simulink model "mc_att_control_xyk"  (R2024b)
settings: Solver=FixedStepAuto  StartTime=0.0  StopTime=10.0  RelTol=1e-3
undefined symbols (not defined in the file or in its folder): AIRMODE_ROLL_PITCH_YAW, deg, DiscIntNeverNeededParam, MC_ACRO_EXPO, MC_ACRO_EXPO_Y, MC_ACRO_P_MAX, MC_ACRO_R_MAX, MC_ACRO_SUPEXPO, MC_ACRO_SUPEXPOY, MC_ACRO_Y_MAX, MC_AIRMODE, MC_BAT_SCALE_EN, MC_MAN_TILT_TAU, MC_PITCH_P, MC_PITCHRATE_D, MC_PITCHRATE_FF, MC_PITCHRATE_I, MC_PITCHRATE_K, MC_PITCHRATE_MAX, MC_PITCHRATE_P, MC_PR_INT_LIM, MC_ROLL_P, MC_ROLLRATE_D, MC_ROLLRATE_FF, MC_ROLLRATE_I, MC_ROLLRATE_K, MC_ROLLRATE_MAX, MC_ROLLRATE_P, MC_RR_INT_LIM, MC_YAW_P, MC_YAW_WEIGHT, MC_YAWRATE_D, MC_YAWRATE_FF, MC_YAWRATE_I, MC_YAWRATE_K, MC_YAWRATE_MAX, MC_YAWRATE_P, MC_YR_INT_LIM, MPC_MAN_TILT_MAX, MPC_MAN_Y_MAX, MPC_MANTHR_MIN, MPC_THR_CURVE, MPC_THR_HOVER, MPC_THR_MAX, param_mpc_thr_hover, param_mpc_thr_max, rad, s, VEHICLE_TYPE_ROTARY_WING
libraries: simulink x22, aerolibutil x11, sharedtransform x4, aerolibconvert2 x3, vrlib x2, sharedutil x1
(part 2 of 2)

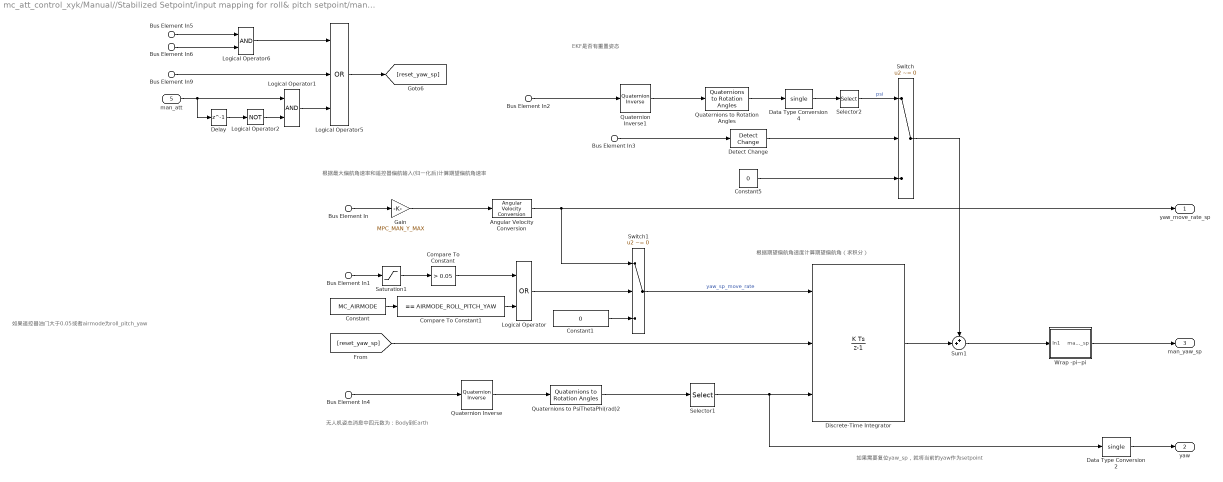
== system mc_att_control_xyk/Manual//Stabilized Setpoint/input mapping for roll& pitch setpoint/man_yaw_sp ==
  note: 无人机姿态消息中四元数为：Body到Earth
  note: 根据期望偏航角速度计算期望偏航角（求积分）
  note: 根据最大偏航角速率和遥控器偏航输入(归一化后)计算期望偏航角速率
  note: 如果遥控器油门大于0.05或者airmode为roll_pitch_yaw
  note: EKF是否有重置姿态
  note: 如果需要复位yaw_sp，就将当前的yaw作为setpoint
  Bus Element In2 : Inport  PortName=att  Element=delta_q_reset
  Bus Element In3 : Inport  PortName=att  Element=quat_reset_counter
  Bus Element In4 : Inport  PortName=att  Element=q
  Bus Element In : Inport  Port=2  PortName=manual_setpoint  Element=r
  Bus Element In1 : Inport  Port=2  PortName=manual_setpoint  Element=z
  Bus Element In5 : Inport  Port=3  PortName=vehicle_status  Element=is_vtol
  Bus Element In6 : Inport  Port=3  PortName=vehicle_status  Element=in_transition_mode
  Bus Element In9 : Inport  Port=4  PortName=vehicle_land_detected  Element=landed
  man_att : Inport  Port=5
  Angular Velocity Conversion : aerolibconvert2/Angular Velocity Conversion  IU=deg/s  OU=rad/s
  Compare To Constant : simulink/Logic and Bit Operations/Compare To Constant  relop=>  const=0.05  OutDataTypeStr=boolean
  Compare To Constant1 : simulink/Logic and Bit Operations/Compare To Constant  relop===  const=AIRMODE_ROLL_PITCH_YAW  OutDataTypeStr=boolean
  Constant : Constant  Value=MC_AIRMODE
  Constant1 : Constant  Value=0  OutDataTypeStr=single
  Constant5 : Constant  Value=0  OutDataTypeStr=single
  Data Type Conversion2 : DataTypeConversion  OutDataTypeStr=single  SaturateOnIntegerOverflow=off  RndMeth=Floor
  Data Type Conversion4 : DataTypeConversion  OutDataTypeStr=single  SaturateOnIntegerOverflow=off  RndMeth=Floor
  Delay : Delay  DelayLength=1  InitialCondition=0
  Detect Change : simulink/Logic and Bit Operations/Detect Change  vinit=0  OutDataTypeStr=boolean
  Discrete-Time Integrator : DiscreteIntegrator  ExternalReset=level  InitialConditionSource=external  SampleTime=-1  LimitOutput=on  UpperSaturationLimit=pi  LowerSaturationLimit=-pi  ICPrevOutput=DiscIntNeverNeededParam  ICPrevScaledInput=DiscIntNeverNeededParam
  Gain : Gain  Gain=MPC_MAN_Y_MAX
      settings: AttributesFormatString=%<Gain>
  Logical Operator : Logic  Operator=OR  AllPortsSameDT=off  OutDataTypeStr=boolean
  Logical Operator1 : Logic  AllPortsSameDT=off  OutDataTypeStr=boolean
  Logical Operator2 : Logic  Operator=NOT  AllPortsSameDT=off  OutDataTypeStr=boolean
  Logical Operator5 : Logic  Operator=OR  Inputs=3  AllPortsSameDT=off  OutDataTypeStr=boolean
  Logical Operator6 : Logic  AllPortsSameDT=off  OutDataTypeStr=boolean
  Quaternion Inverse : aerolibutil/Quaternion Inverse
  Quaternion Inverse1 : aerolibutil/Quaternion Inverse
  Quaternions to PsiThetaPhi(rad)2 : sharedtransform/Quaternions to Rotation Angles  rotationOrder=ZYX  aMode=aMode
  Quaternions to Rotation Angles : sharedtransform/Quaternions to Rotation Angles  rotationOrder=ZYX  aMode=aMode
  Saturation1 : Saturate  UpperLimit=1  LowerLimit=0
      settings: AttributesFormatString=[%<LowerLimit>,%<UpperLimit>]
  Selector1 : Selector  InputPortWidth=3  IndexOptions=Index vector (dialog)  Indices=1  OutputSizes=1
  Selector2 : Selector  InputPortWidth=3  IndexOptions=Index vector (dialog)  Indices=1  OutputSizes=1
  Sum1 : Sum  Inputs=++|
  Switch : Switch  Criteria=u2 ~= 0  SaturateOnIntegerOverflow=off  InputSameDT=off
  Switch1 : Switch  Criteria=u2 ~= 0  SaturateOnIntegerOverflow=off  InputSameDT=off
  Wrap -pi~pi : Subsystem
  yaw_move_rate_sp : Outport
  yaw : Outport  Port=2
  man_yaw_sp : Outport  Port=3
  wires:
  Quaternions to PsiThetaPhi(rad)2/1 -> Selector1/1
  Quaternions to Rotation Angles/1 -> Data Type Conversion4/1
  Constant5/1 -> Switch/3
  Detect Change/1 -> Switch/2
  Gain/1 -> Angular Velocity Conversion/1
  Switch/1 -> Sum1/1
  Sum1/1 -> Wrap -pi~pi/1(In1)
  Selector1/1 -> Data Type Conversion2/1, Discrete-Time Integrator/3
  Angular Velocity Conversion/1 -> yaw_move_rate_sp/1, Switch1/1
  Discrete-Time Integrator/1 -> Sum1/2
  Selector2/1 -> Switch/1  "psi"
  [reset_yaw_sp] -> Discrete-Time Integrator/2
  Bus Element In/1 -> Gain/1
  Bus Element In3/1 -> Detect Change/1
  Switch1/1 -> Discrete-Time Integrator/1  "yaw_sp_move_rate"
  Bus Element In1/1 -> Saturation1/1
  Saturation1/1 -> Compare To Constant/1
  Compare To Constant/1 -> Logical Operator/1
  Constant/1 -> Compare To Constant1/1
  Logical Operator/1 -> Switch1/2
  Compare To Constant1/1 -> Logical Operator/2
  Logical Operator6/1 -> Logical Operator5/1
  Bus Element In6/1 -> Logical Operator6/2
  Logical Operator5/1 -> [reset_yaw_sp]
  Bus Element In9/1 -> Logical Operator5/2
  Bus Element In5/1 -> Logical Operator6/1
  Logical Operator1/1 -> Logical Operator5/3
  man_att/1 -> Delay/1, Logical Operator1/1
  Logical Operator2/1 -> Logical Operator1/2
  Delay/1 -> Logical Operator2/1
  Bus Element In4/1 -> Quaternion Inverse/1
  Bus Element In2/1 -> Quaternion Inverse1/1
  Data Type Conversion4/1 -> Selector2/1
  Quaternion Inverse/1 -> Quaternions to PsiThetaPhi(rad)2/1
  Quaternion Inverse1/1 -> Quaternions to Rotation Angles/1
  Constant1/1 -> Switch1/3
  Wrap -pi~pi/1(man_yaw_sp) -> man_yaw_sp/1
  Data Type Conversion2/1 -> yaw/1

== system mc_att_control_xyk/Manual//Stabilized Setpoint/input mapping for roll& pitch setpoint/vector limitation ==
  v : Inport
  Divide : Product  Inputs=*/
  Dot Product2 : DotProduct  OutDataTypeStr=Inherit: Inherit via internal rule
  Gain : Gain  Gain=MPC_MAN_TILT_MAX
      settings: AttributesFormatString=%<Gain>
  Sqrt1 : Sqrt
  Switch1 : Switch  Criteria=u2 > Threshold  Threshold=MPC_MAN_TILT_MAX  SaturateOnIntegerOverflow=off  InputSameDT=off
  v_limited : Outport
  wires:
  Switch1/1 -> v_limited/1
  Dot Product2/1 -> Sqrt1/1
  Sqrt1/1 -> Switch1/2, Divide/2  "v_norm"
  Divide/1 -> Gain/1
  v/1 -> Divide/1, Switch1/3, Dot Product2/2, Dot Product2/1
  Gain/1 -> Switch1/1

== system mc_att_control_xyk/Manual//Stabilized Setpoint/vtol modify roll//pitch/Wrap -pi~pi ==
  In1 : Inport
  Constant1 : Constant  Value=2*pi  OutDataTypeStr=single
  Mod : Math  Operator=mod
  Sum1 : Sum  Inputs=|+-
  Switch : Switch  Criteria=u2 > Threshold  Threshold=pi  SaturateOnIntegerOverflow=off  InputSameDT=off
  Out1 : Outport
  wires:
  Sum1/1 -> Switch/1
  Mod/1 -> Switch/3, Sum1/1, Switch/2
  Constant1/1 -> Sum1/2, Mod/2
  Switch/1 -> Out1/1
  In1/1 -> Mod/1

== system mc_att_control_xyk/Rate Control/I/mixer saturation ==
  rate_err : Inport
  Bitwise Operator : simulink/Logic and Bit Operations/Bitwise Operator  logicop=AND  UseBitMask=on  BitMask=bin2dec('00001000')  BitMaskRealWorld=Stored Integer
  Bitwise Operator1 : simulink/Logic and Bit Operations/Bitwise Operator  logicop=AND  UseBitMask=on  BitMask=bin2dec('00010000')  BitMaskRealWorld=Stored Integer
  Bitwise Operator2 : simulink/Logic and Bit Operations/Bitwise Operator  logicop=AND  UseBitMask=on  BitMask=bin2dec('00100000')  BitMaskRealWorld=Stored Integer
  Bitwise Operator3 : simulink/Logic and Bit Operations/Bitwise Operator  logicop=AND  UseBitMask=on  BitMask=bin2dec('01000000')  BitMaskRealWorld=Stored Integer
  Bitwise Operator4 : simulink/Logic and Bit Operations/Bitwise Operator  logicop=AND  UseBitMask=on  BitMask=bin2dec('10000000')  BitMaskRealWorld=Stored Integer
  Bitwise Operator5 : simulink/Logic and Bit Operations/Bitwise Operator  logicop=AND  UseBitMask=on  BitMask=bin2dec('100000000')  BitMaskRealWorld=Stored Integer
  Compare To Constant : simulink/Logic and Bit Operations/Compare To Constant  relop=>=  const=0.0  OutDataTypeStr=boolean
  Compare To Constant1 : simulink/Logic and Bit Operations/Compare To Constant  relop=<  const=0.0  OutDataTypeStr=boolean
  Constant : Constant  Value=[0 0 0]  OutDataTypeStr=single
  Logical Operator : Logic  AllPortsSameDT=off  OutDataTypeStr=boolean
  Logical Operator1 : Logic  AllPortsSameDT=off  OutDataTypeStr=boolean
  Logical Operator2 : Logic  Operator=OR  AllPortsSameDT=off  OutDataTypeStr=boolean
  Mux : Mux  Inputs=3
  Mux1 : Mux  Inputs=3
  Switch : Switch  Criteria=u2 ~= 0  SaturateOnIntegerOverflow=off  InputSameDT=off
  rate_err1 : InportShadow
  rate_err_limited : Outport
  wires:
  [saturation_status] -> Bitwise Operator5/1, Bitwise Operator3/1, Bitwise Operator1/1, Bitwise Operator/1, Bitwise Operator2/1, Bitwise Operator4/1
  Bitwise Operator/1 -> Mux/1  "roll_pos"
  Bitwise Operator1/1 -> Mux1/1  "roll_neg"
  Bitwise Operator2/1 -> Mux/2  "pitch_pos"
  Bitwise Operator3/1 -> Mux1/2  "pitch_neg"
  Bitwise Operator4/1 -> Mux/3  "yaw_pos"
  Bitwise Operator5/1 -> Mux1/3  "yaw_neg"
  Mux/1 -> [pos]
  Mux1/1 -> [neg]
  Compare To Constant/1 -> Logical Operator/2
  rate_err/1 -> Compare To Constant/1, Compare To Constant1/1
  [pos] -> Logical Operator/1
  [neg] -> Logical Operator1/2
  Compare To Constant1/1 -> Logical Operator1/1
  Logical Operator/1 -> Logical Operator2/1
  Logical Operator1/1 -> Logical Operator2/2
  Logical Operator2/1 -> Switch/2
  Constant/1 -> Switch/1
  rate_err1/1 -> Switch/3
  Switch/1 -> rate_err_limited/1

== system mc_att_control_xyk/Manual//Stabilized Setpoint/input mapping for roll& pitch setpoint/man_yaw_sp/Wrap -pi~pi ==
  In1 : Inport
  Bias : Bias  Bias=pi  SaturateOnIntegerOverflow=off
  Bias1 : Bias  Bias=-pi  SaturateOnIntegerOverflow=off
  Constant1 : Constant  Value=2*pi  OutDataTypeStr=single
  Mod : Math  Operator=mod
  man_yaw_sp : Outport
  wires:
  Constant1/1 -> Mod/2
  Mod/1 -> Bias1/1
  In1/1 -> Bias/1
  Bias/1 -> Mod/1
  Bias1/1 -> man_yaw_sp/1
